simulink model "rising_edge_Counter"  (R2023a)
settings: Solver=FixedStepAuto  StartTime=0.0  StopTime=50  RelTol=1e-3
settings Model: Creator=EMRIX  LastModifiedBy=EMRIX

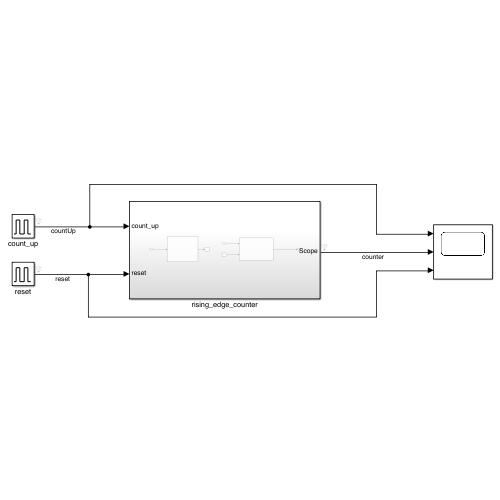
[thumbnail: Simulink's stored preview of the top-level diagram]
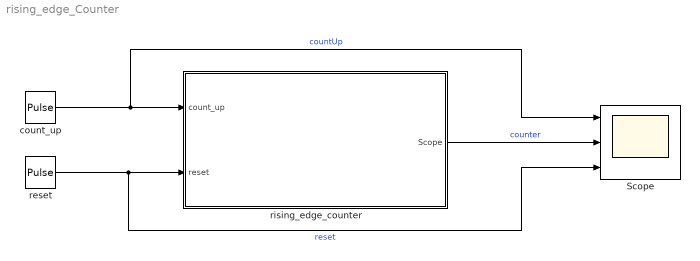
== system rising_edge_Counter ==
  Scope : Scope  NumInputPorts=3
  count_up : DiscretePulseGenerator  PulseType=Time based  PulseWidth=5
  reset : DiscretePulseGenerator  PulseType=Time based  Period=20  PulseWidth=20
  rising_edge_counter : Subsystem
  wires:
  reset/1 -> Scope/3, rising_edge_counter/2(reset)  "reset"
  count_up/1 -> rising_edge_counter/1(count_up), Scope/1  "countUp"
  rising_edge_counter/1(Scope) -> Scope/2  "counter"

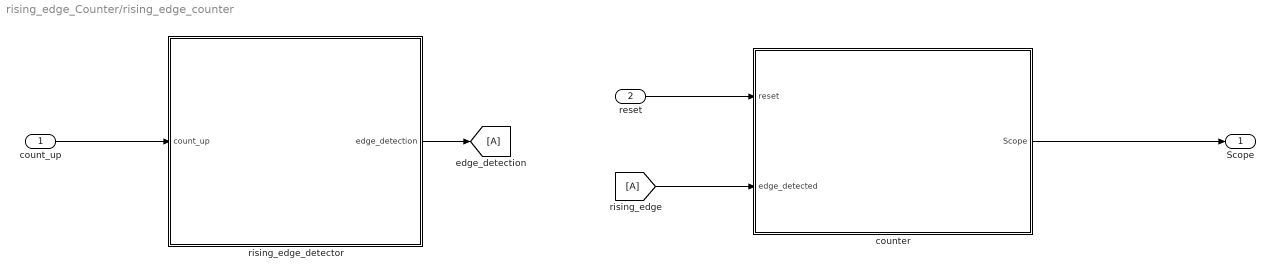
== system rising_edge_Counter/rising_edge_counter ==
  count_up : Inport
  reset : Inport  Port=2
  counter : Subsystem
  edge_detection : Goto
  rising_edge : From
  rising_edge_detector : Subsystem
  Scope : Outport
  wires:
  count_up/1 -> rising_edge_detector/1(count_up)
  rising_edge_detector/1(edge_detection) -> edge_detection/1
  reset/1 -> counter/1(reset)
  counter/1(Scope) -> Scope/1
  rising_edge/1 -> counter/2(edge_detected)

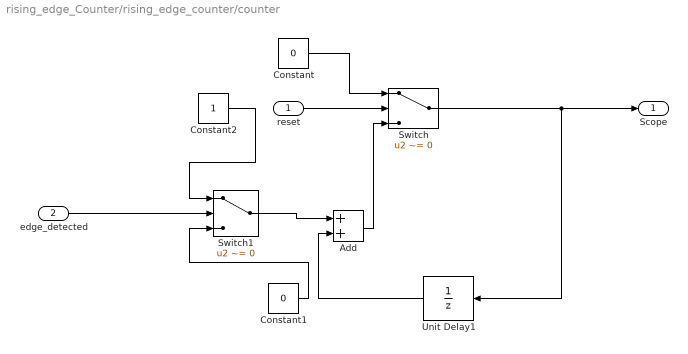
== system rising_edge_Counter/rising_edge_counter/counter ==
  reset : Inport
  edge_detected : Inport  Port=2
  Add : Sum
  Constant : Constant  Value=0
  Constant1 : Constant  Value=0
  Constant2 : Constant
  Switch : Switch  Criteria=u2 ~= 0  SaturateOnIntegerOverflow=off  InputSameDT=off
  Switch1 : Switch  Criteria=u2 ~= 0  SaturateOnIntegerOverflow=off  InputSameDT=off
  Unit Delay1 : UnitDelay  SampleTime=-1  HasFrameUpgradeWarning=on
  Scope : Outport
  wires:
  Switch/1 -> Scope/1, Unit Delay1/1
  Add/1 -> Switch/3
  Switch1/1 -> Add/1
  reset/1 -> Switch/2
  Constant/1 -> Switch/1
  Unit Delay1/1 -> Add/2
  Constant2/1 -> Switch1/1
  Constant1/1 -> Switch1/3
  edge_detected/1 -> Switch1/2

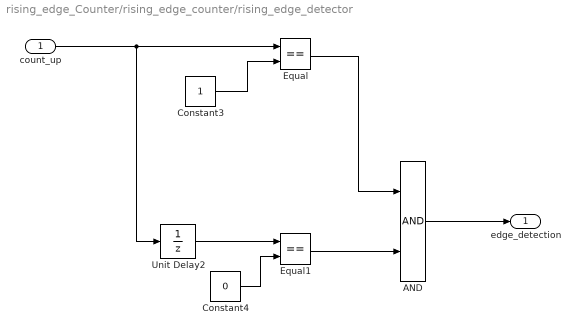
== system rising_edge_Counter/rising_edge_counter/rising_edge_detector ==
  count_up : Inport
  AND : Logic  AllPortsSameDT=off  OutDataTypeStr=boolean
  Constant3 : Constant
  Constant4 : Constant  Value=0
  Equal : RelationalOperator  Operator===  OutDataTypeStr=boolean  RndMeth=Simplest  InputSameDT=off
  Equal1 : RelationalOperator  Operator===  OutDataTypeStr=boolean  RndMeth=Simplest  InputSameDT=off
  Unit Delay2 : UnitDelay  SampleTime=-1  HasFrameUpgradeWarning=on
  edge_detection : Outport
  wires:
  AND/1 -> edge_detection/1
  Equal1/1 -> AND/2
  count_up/1 -> Unit Delay2/1, Equal/1
  Constant4/1 -> Equal1/2
  Constant3/1 -> Equal/2
  Unit Delay2/1 -> Equal1/1
  Equal/1 -> AND/1
